simulink model "Teleoperation_Task_Space"  (R2021b)
settings: Solver=FixedStepAuto  StartTime=0.0  StopTime=20  FixedStep=Ts  RelTol=1e-3
values from neighbouring files (symbols this model uses):
  alphas_m = 25.0 * ones(1,dh.dof)    [setup_teleop.m]
  alphas_s = 16.5 * ones(1,dh.dof)    [setup_teleop.m]
  B_m = diag(ones(1,dh.dof)) * 32    [setup_teleop.m]
  B_s = diag(ones(1,dh.dof)) * 4    [setup_teleop.m]
  fc_in = 0.8    [setup_teleop.m]
  gravity = [0 0 9.81]'    [setup_robot.m]
  K_g = eye(dh.dof) * k_g    [setup_teleop.m]
  K_m = diag(ones(1,dh.dof)) * 22    [setup_teleop.m]
  K_s = diag(ones(1,dh.dof)) * 4    [setup_teleop.m]
  lambdas_m = 7.5 * ones(1,dh.dof)    [setup_teleop.m]
  lambdas_s = 3.0 * ones(1,dh.dof)    [setup_teleop.m]
  M_m = diag(ones(1,dh.dof)) * 22    [setup_teleop.m]
  M_s = diag(ones(1,dh.dof)) * 1    [setup_teleop.m]
  T_m2s = 25 / 1000 / Ts    (= 25)    [setup_teleop.m]
  T_s2m = 25 / 1000 / Ts    (= 25)    [setup_teleop.m]
  zdq_A = [1 3*wc 3*wc^2 wc^3]    [setup_teleop.m]
  zdq_B = [0 0 0 wc^3]    [setup_teleop.m]
undefined symbols (not defined in the file or in its folder): conf, dh, Fm_A, Fm_B, Fs_A, Fs_B, G, sigbuilder_block, x0
libraries: simulink x2, vrlib x2
(part 2 of 2)

== matlab function Teleoperation_Task_Space/Slave Observer and Force Estimator/Injectable Robot Model (Joint Space)/MATLAB Function3 ==
  data: dh parameter; dX output; q input; dq input
function dX = JA(dh, q, dq)
    dX = JA_rne(dh, q)*dq;
end

== matlab function Teleoperation_Task_Space/Slave Observer and Force Estimator/Injectable Robot Model (Joint Space)/MATLAB Function4 ==
  data: q input size=dh.dof; inject_ddq output size=dh.dof; inject_ddX input size=2; dh parameter
function inject_ddq = get_inject_ddq(q, inject_ddX, dh)
    JA = JA_rne(dh, q);
    inject_ddq = pinv(JA) * inject_ddX;
end

== matlab function Teleoperation_Task_Space/Slave Observer and Force Estimator/Injectable Robot Model (Joint Space)/MATLAB Function5 ==
  data: q input size=dh.dof; inject_dq output size=dh.dof; inject_dX input size=2; dh parameter
function inject_dq = get_inject_dq(q, inject_dX, dh)
    JA = JA_rne(dh, q);
    inject_dq = pinv(JA) * inject_dX;
end

== matlab function Teleoperation_Task_Space/Slave Observer and Force Estimator/MATLAB Function1 ==
  data: Fe output; q input; zs2eq input; dh parameter
function Fe = BA_zm(q, zs2eq, dh)
     BA = BA_rne(dh, q);
     Fe = - BA * zs2eq;
end

== matlab function Teleoperation_Task_Space/Slave Observer and Force Estimator/Injectable Robot Model (Joint Space)/MATLAB Function ==
  data ddq_ settings: updateMethod=SF_CONTINUOUS_TIME_DATA
  data dq_ settings: updateMethod=SF_CONTINUOUS_TIME_DATA
  data dq settings: updateMethod=SF_CONTINUOUS_TIME_DATA
  data q settings: updateMethod=SF_CONTINUOUS_TIME_DATA
  data u settings: updateMethod=SF_CONTINUOUS_TIME_DATA
  data: ddq_ output size=dh.dof; dq_ output size=dh.dof; dq input size=dh.dof; q input size=dh.dof; u input size=dh.dof; g input size=3; dh parameter
function [ddq_, dq_]  = RobotSystem(dq, q, u, g, dh)
    
    % compute dynamics
    B = B_rne(dh, q);
    C = C_rne(dh, q, dq);
    G = G_rne(dh, q, g);

    dq_ = dq(1:dh.dof);

    ddq = B \ (u - C*dq - G);
    ddq_ = ddq(1:dh.dof);
end

== matlab function Teleoperation_Task_Space/Slave Observer and Force Estimator/Injectable Robot Model (Joint Space)/MATLAB Function1 ==
  data: X output; q input; dh parameter
function X = K(q, dh)
    X = K_rne(dh, q);
end

== matlab function Teleoperation_Task_Space/Slave controller/Slave Controller ==
  data: dh parameter; gravity parameter size=3; qs input size=dh.dof; dqs input size=dh.dof; Xs input size=2; Fs output size=2; dXs input size=2; qm input size=dh.dof; Xm input size=2; dXm input size=2; Fh input size=2; Fe input size=2; Fedd input size=2; zs2eq input size=2; zm2eq input size=2; sign_s input size=2; M_m parameter size=[2,2]; B_m parameter size=[2,2]; K_m parameter size=[2,2]; M_s parameter size=[2,2]; B_s parameter size=[2,2]; K_s parameter size=[2,2]; K_g parameter size=[2,2]
function Fs = Cs(dh,gravity, qs,dqs,Xs,dXs, qm,Xm,dXm, Fh,Fe,Fedd, zs2eq,zm2eq,sign_s, M_m,B_m,K_m, M_s,B_s,K_s,K_g)

    MAs = BA_rne(dh, qs);
    if any(~isfinite(MAs))
        MAs = zeros(size(MAs));
    end
    CAdX = CAdX_rne(dh, qs, dqs);
    GAs = GA_rne(dh, qs, gravity);
    hAs = CAdX + GAs;
    % TODO needs the master dh, but in this project we have the same robots
    MAm = BA_rne(dh, qm);
    if any(~isfinite(MAm))
        MAm = zeros(size(MAm));
    end
    
    Fs = -MAs * (M_s\K_s*Xs + M_s\B_s*dXs ...
                - MAs\hAs ...
                + (M_m\K_m - M_s\K_s)*Xm ...
                + (M_m\B_m - M_s\B_s)*dXm ...
                - (inv(M_m) - pinv(MAm))*Fh ...
                + M_m\Fedd + M_s\Fe ...
                + zs2eq + zm2eq + K_g*sign_s);
    Fs = Fs;
end

== matlab function Teleoperation_Task_Space/MATLAB Function ==
  data: X input; he input; hA output
function hA = TAT(X,he)
    hA = TA(X)' * he;
end

== matlab function Teleoperation_Task_Space/Master Robot/Injectable Robot Model (Joint Space)/MATLAB Function ==
  data ddq_ settings: updateMethod=SF_CONTINUOUS_TIME_DATA
  data dq_ settings: updateMethod=SF_CONTINUOUS_TIME_DATA
  data dq settings: updateMethod=SF_CONTINUOUS_TIME_DATA
  data q settings: updateMethod=SF_CONTINUOUS_TIME_DATA
  data u settings: updateMethod=SF_CONTINUOUS_TIME_DATA
  data: ddq_ output size=dh.dof; dq_ output size=dh.dof; dq input size=dh.dof; q input size=dh.dof; u input size=dh.dof; g input size=3; dh parameter
function [ddq_, dq_]  = RobotSystem(dq, q, u, g, dh)
    
    % compute dynamics
    B = B_rne(dh, q);
    C = C_rne(dh, q, dq);
    G = G_rne(dh, q, g);

    dq_ = dq(1:dh.dof);

    ddq = B \ (u - C*dq - G);
    ddq_ = ddq(1:dh.dof);
end
